simulink model "CRA_Assignment5"  (R2022b)
settings: Solver=ode23  StartTime=0.0  StopTime=1800  RelTol=1e-7  AbsTol=1e-7
settings Model: Creator=lerio  LastModifiedBy=lerio

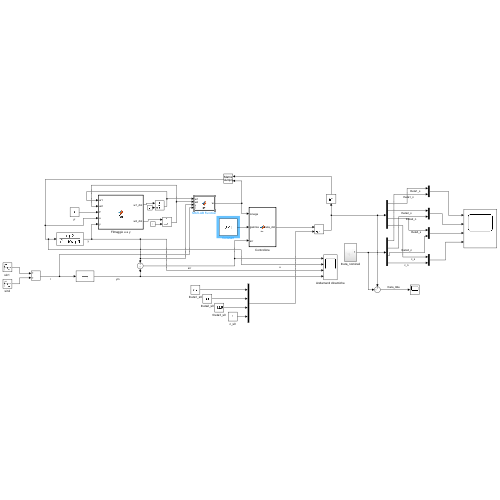
[thumbnail: Simulink's stored preview of the top-level diagram]
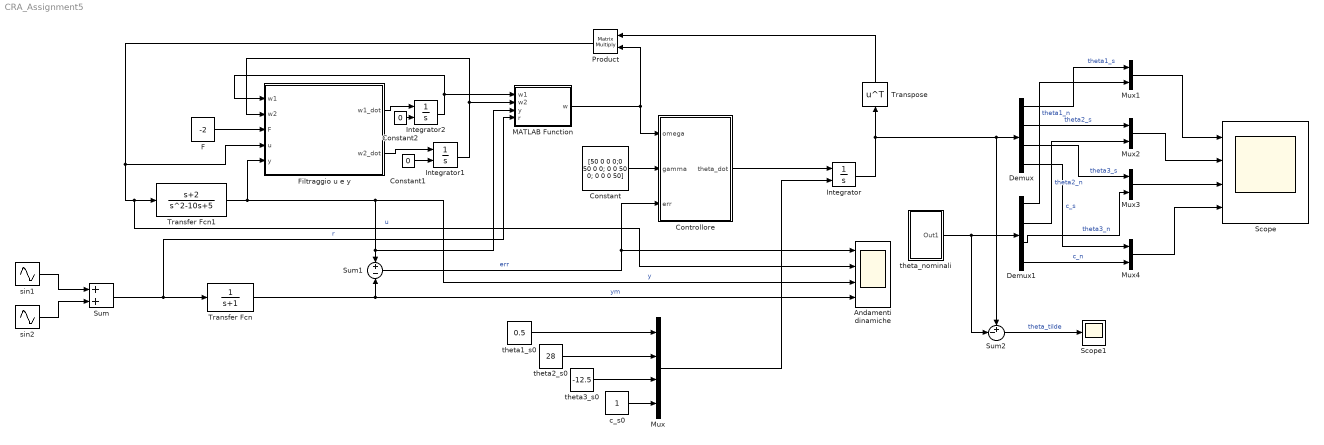
== system CRA_Assignment5 ==
  Andamenti dinamiche : Scope  NumInputPorts=4
  Constant : Constant  Value=[50 0 0 0;0 50 0 0; 0 0 50 0; 0 0 0 50]  VectorParams1D=off
  Constant1 : Constant  Value=0
  Constant2 : Constant  Value=0
  Controllore : MATLAB Function  TreatAsAtomicUnit=on
  Demux : Demux
  Demux1 : Demux
  F : Constant  Value=-2
  Filtraggio u e y : MATLAB Function  TreatAsAtomicUnit=on
  Integrator : Integrator  InitialConditionSource=external
  Integrator1 : Integrator  InitialConditionSource=external  InitialCondition=70
  Integrator2 : Integrator  InitialConditionSource=external  InitialCondition=40
  MATLAB Function : MATLAB Function  TreatAsAtomicUnit=on
  Mux : Mux
  Mux{1..4} (4 alike) : Mux  Inputs=2
  Product : Product  Multiplication=Matrix(*)
  Scope : Scope  NumInputPorts=4
  Scope1 : Scope
  Sum : Sum
  Sum1 : Sum  Inputs=+-
  Sum2 : Sum  Inputs=+-|
  Transfer Fcn : TransferFcn  Denominator=[1 1]
  Transfer Fcn1 : TransferFcn  Numerator=[1 2]  Denominator=[1 -10 5]
  Transpose : Math  Operator=transpose
  c_s0 : Constant
  "sin1 " : Sin  Amplitude=0.5  Frequency=10  SampleTime=0
  sin2 : Sin  Amplitude=5  Frequency=0.1  SampleTime=0
  theta1_s0 : Constant  Value=0.5
  theta2_s0 : Constant  Value=28
  theta3_s0 : Constant  Value=-12.5
  theta_nominali : Subsystem
  wires:
  "sin1 "/1 -> Sum/1
  sin2/1 -> Sum/2
  Sum/1 -> MATLAB Function/4(r), Transfer Fcn/1  "r"
  Transfer Fcn/1 -> Sum1/2, Andamenti dinamiche/4  "ym"
  Sum1/1 -> Controllore/3(err), Andamenti dinamiche/1  "err"
  Filtraggio u e y/2(w2_dot) -> Integrator1/1
  Integrator1/1 -> MATLAB Function/2(w2), Filtraggio u e y/2(w2)
  Transfer Fcn1/1 -> Filtraggio u e y/5(y), Andamenti dinamiche/3, MATLAB Function/3(y), Sum1/1  "y"
  F/1 -> Filtraggio u e y/3(F)
  Filtraggio u e y/1(w1_dot) -> Integrator2/1
  Integrator2/1 -> MATLAB Function/1(w1), Filtraggio u e y/1(w1)
  MATLAB Function/1(w) -> Controllore/1(omega), Product/2
  Constant/1 -> Controllore/2(gamma)
  Controllore/1(theta_dot) -> Integrator/1
  Product/1 -> Andamenti dinamiche/2, Transfer Fcn1/1, Filtraggio u e y/4(u)  "u"
  Transpose/1 -> Product/1
  theta1_s0/1 -> Mux/1
  theta2_s0/1 -> Mux/2
  theta3_s0/1 -> Mux/3
  c_s0/1 -> Mux/4
  Mux/1 -> Integrator/2
  theta_nominali/1(Out1) -> Sum2/2, Demux1/1
  Demux/1 -> Mux1/1  "theta1_s"
  Demux1/1 -> Mux1/2  "theta1_n"
  Demux1/2 -> Mux2/2  "theta2_n"
  Demux/2 -> Mux2/1  "theta2_s"
  Demux/3 -> Mux3/1  "theta3_s"
  Demux1/3 -> Mux3/2  "theta3_n"
  Demux/4 -> Mux4/1  "c_s"
  Demux1/4 -> Mux4/2  "c_n"
  Mux1/1 -> Scope/1
  Mux2/1 -> Scope/2
  Mux3/1 -> Scope/3
  Mux4/1 -> Scope/4
  Sum2/1 -> Scope1/1  "theta_tilde"
  Integrator/1 -> Transpose/1, Sum2/1, Demux/1
  Constant1/1 -> Integrator1/2
  Constant2/1 -> Integrator2/2

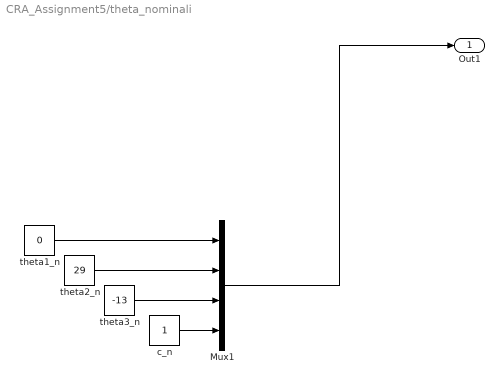
== system CRA_Assignment5/theta_nominali ==
  Mux1 : Mux
  c_n : Constant
  theta1_n : Constant  Value=0
  theta2_n : Constant  Value=29
  theta3_n : Constant  Value=-13
  Out1 : Outport
  wires:
  Mux1/1 -> Out1/1
  c_n/1 -> Mux1/4
  theta1_n/1 -> Mux1/1
  theta3_n/1 -> Mux1/3
  theta2_n/1 -> Mux1/2

== matlab function CRA_Assignment5/Filtraggio u e y ==
  data: w1 input; w1_dot output; w2 input; F input; u input; y input; w2_dot output
function [w1_dot,w2_dot] = fcn(w1,w2,F,u,y)

w1_dot = F*w1+u;
w2_dot = F*w2+y;

== matlab function CRA_Assignment5/MATLAB Function ==
  data: w1 input; w output; w2 input; y input; r input
function w = fcn(w1,w2,y,r)

w = [w1;w2;y;r];

== matlab function CRA_Assignment5/Controllore ==
  data: omega input; gamma input; theta_dot output; err input
function theta_dot = fcn(omega,gamma,err)

theta_dot = -gamma*err*omega;
